simulink model "inputs"  (R2017a)
settings: Solver=FixedStepDiscrete  StartTime=0.0  StopTime=10.0  FixedStep=1  RelTol=1e-3
settings Model: Creator=ptracton  LastModifiedBy=ptracton

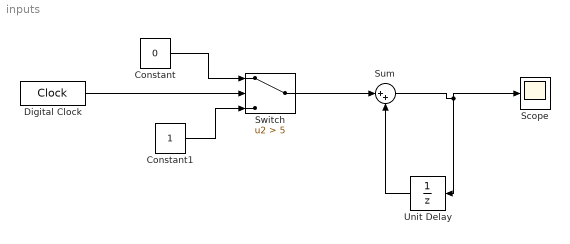
== system inputs ==
  Constant : Constant  Value=0
  Constant1 : Constant
  Digital Clock : DigitalClock
  Scope : Scope
  Sum : Sum  Inputs=|++
  Switch : Switch  Criteria=u2 > Threshold  Threshold=5
  Unit Delay : UnitDelay  SampleTime=-1
  wires:
  Digital Clock/1 -> Switch/2
  Constant1/1 -> Switch/3
  Constant/1 -> Switch/1
  Switch/1 -> Sum/1
  Sum/1 -> Unit Delay/1, Scope/1
  Unit Delay/1 -> Sum/2
